simulink model "test_thrustflapping"  (Simulink 7.7)
settings: Solver=ode45  StartTime=0.0  StopTime=10  RelTol=1e-3
settings Model: Creator=Administrator  LastModifiedBy=Administrator
settings DataIOCC: LimitDataPoints=off  LoadExternalInput=on  OutputSaveName=T_MR

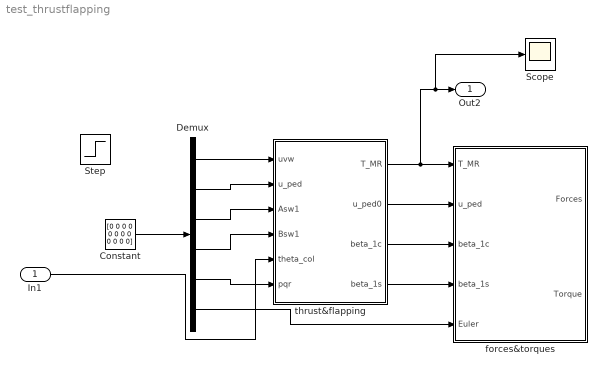
== system test_thrustflapping ==
  In1 : Inport
  Constant : Constant  Value=[0 0 0 0 0 0 0 0 0 0 0 0]
  Demux : Demux  Outputs=[3 1 1 1 3 3]
  Scope : Scope
  Step : Step  Time=0.5  After=0.5  SampleTime=0
  forces&torques : Subsystem  mask{mass0=44.384, AQ=0.00036, BQ=0.01, lm=0, ym=0, hm=0.2, Lt=1.2, Ht=0}
  thrust&flapping : Subsystem  mask{Ksw=0.2, Kcr=0.8, T_old=10, vi0=5, theta_twist=4.864e-4, theta_0=0.07}
  Out2 : Outport
  wires:
  Constant/1 -> Demux/1
  thrust&flapping/1(T_MR) -> forces&torques/1(T_MR), Out2/1, Scope/1
  thrust&flapping/2(u_ped0) -> forces&torques/2(u_ped)
  thrust&flapping/3(beta_1c) -> forces&torques/3(beta_1c)
  thrust&flapping/4(beta_1s) -> forces&torques/4(beta_1s)
  Demux/1 -> thrust&flapping/1(uvw)
  Demux/2 -> thrust&flapping/2(u_ped)
  Demux/3 -> thrust&flapping/3(Asw1)
  Demux/4 -> thrust&flapping/4(Bsw1)
  Demux/5 -> thrust&flapping/6(pqr)
  Demux/6 -> forces&torques/5(Euler)
  In1/1 -> thrust&flapping/5(theta_col)

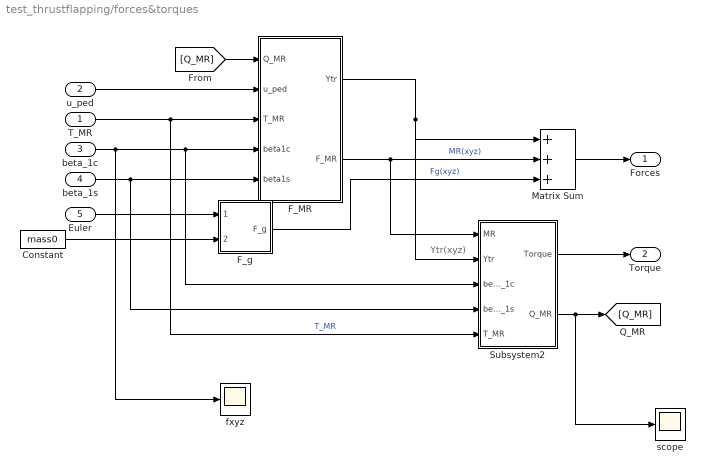
== system test_thrustflapping/forces&torques ==
  note: Ytr(xyz)
  T_MR : Inport
  u_ped : Inport  Port=2
  beta_1c : Inport  Port=3
  beta_1s : Inport  Port=4
  Euler : Inport  Port=5
  Constant : Constant  Value=mass0
  F_MR : Subsystem
  F_g : Subsystem
  Matrix Sum : Sum  Inputs=+++  CollapseMode=Specified dimension  CollapseDim=3
  Subsystem2 : Subsystem
  fxyz : Scope
      settings: YMin=-37.5  YMax=10  SaveName=ScopeData9
  scope : Scope
      settings: YMin=-37.5  YMax=10  SaveName=ScopeData14
  Forces : Outport
  Torque : Outport  Port=2
  wires:
  F_MR/1(Ytr) -> Subsystem2/2(Ytr), Matrix Sum/1
  u_ped/1 -> F_MR/2(u_ped)
  Matrix Sum/1 -> Forces/1
  Subsystem2/1(Torque) -> Torque/1
  Constant/1 -> F_g/2(mass)
  F_g/1(F_g) -> Matrix Sum/3  "Fg(xyz)"
  Euler/1 -> F_g/1(Euler)
  T_MR/1 -> Subsystem2/5(T_MR), F_MR/3(T_MR)  "T_MR"
  Subsystem2/2(Q_MR) -> [Q_MR], scope/1
  [Q_MR] -> F_MR/1(Q_MR)
  beta_1c/1 -> F_MR/4(beta1c), Subsystem2/3(beta_1c), fxyz/1
  beta_1s/1 -> F_MR/5(beta1s), Subsystem2/4(beta_1s)
  F_MR/2(F_MR) -> Subsystem2/1(MR), Matrix Sum/2  "MR(xyz)"

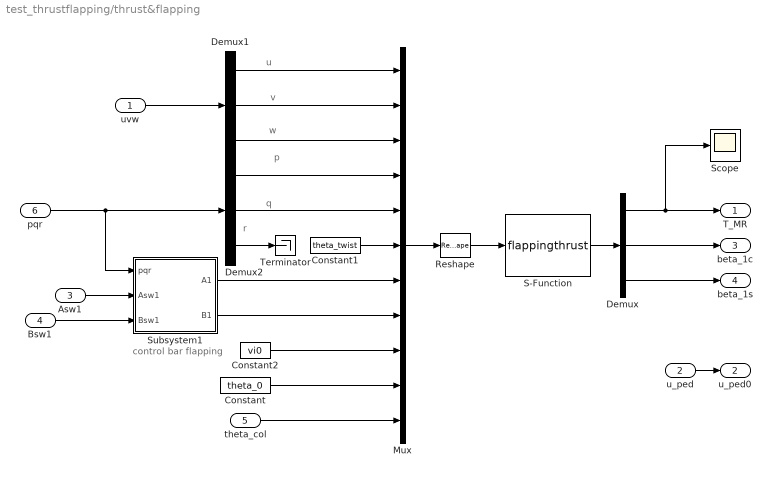
== system test_thrustflapping/thrust&flapping ==
  note: p
  note: q
  note: r
  note: u
  note: v
  note: w
  note: control bar flapping
  uvw : Inport
  u_ped : Inport  Port=2
  Asw1 : Inport  Port=3
  Bsw1 : Inport  Port=4
  theta_col : Inport  Port=5
  pqr : Inport  Port=6
  Constant : Constant  Value=theta_0
  Constant1 : Constant  Value=theta_twist
  Constant2 : Constant  Value=vi0
  Demux : Demux  Outputs=3
  Demux1 : Demux  Outputs=[1 1 1 ]
  Demux2 : Demux  Outputs=[1 1 1]
  Mux : Mux  Inputs=11
  Reshape : Reshape  OutputDimensionality=Column vector (2-D)
  S-Function : S-Function  RequirementInfo={} %GIDa_ec7bf881_92c1_4c8a_a396_57482acf355c  FunctionName=flappingthrust  EnableBusSupport=off
  Scope : Scope
      settings: SaveName=ScopeData4
  Subsystem1 : Subsystem
  Terminator : Terminator
  T_MR : Outport
  u_ped0 : Outport  Port=2
  beta_1c : Outport  Port=3
  beta_1s : Outport  Port=4
  wires:
  u_ped/1 -> u_ped0/1
  S-Function/1 -> Demux/1
  Demux/1 -> T_MR/1, Scope/1
  Demux/2 -> beta_1c/1
  Demux1/1 -> Mux/1
  Demux1/2 -> Mux/2
  Demux1/3 -> Mux/3
  uvw/1 -> Demux1/1
  Demux2/1 -> Mux/4
  Demux2/2 -> Mux/5
  pqr/1 -> Demux2/1, Subsystem1/1(pqr)
  Constant2/1 -> Mux/9
  Demux/3 -> beta_1s/1
  Constant/1 -> Mux/10
  Mux/1 -> Reshape/1
  Reshape/1 -> S-Function/1
  Asw1/1 -> Subsystem1/2(Asw1)
  Bsw1/1 -> Subsystem1/3(Bsw1)
  Subsystem1/1(A1) -> Mux/7
  Subsystem1/2(B1) -> Mux/8
  theta_col/1 -> Mux/11
  Demux2/3 -> Terminator/1
  Constant1/1 -> Mux/6

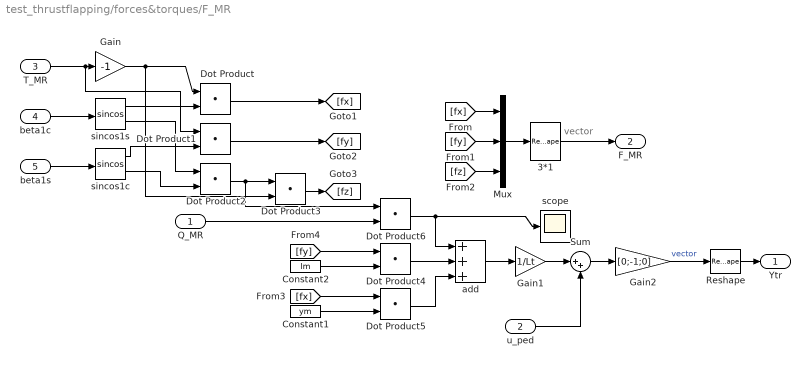
== system test_thrustflapping/forces&torques/F_MR ==
  note: vector
  Q_MR : Inport
  u_ped : Inport  Port=2
  T_MR : Inport  Port=3
  beta1c : Inport  Port=4
  beta1s : Inport  Port=5
  3*1 : Reshape  OutputDimensionality=Column vector (2-D)
  Constant1 : Constant  Value=ym
  Constant2 : Constant  Value=lm
  Dot Product{,1..6} (7 alike) : DotProduct  InputSameDT=on  OutDataTypeStr=Inherit: Inherit via internal rule
  Gain : Gain  Gain=-1
  Gain1 : Gain  Gain=1/Lt
  Gain2 : Gain  Gain=[0;-1;0]
  Mux : Mux  Inputs=3
  Reshape : Reshape  OutputDimensionality=Column vector (2-D)
  Sum : Sum  Inputs=|++
  add : Sum  Inputs=+++
  scope : Scope
      settings: YMin=-37.5  YMax=10  SaveName=ScopeData15
  sincos1c : Trigonometry  Operator=sincos
  sincos1s : Trigonometry  Operator=sincos
  Ytr : Outport
  F_MR : Outport  Port=2
  wires:
  u_ped/1 -> Sum/2
  Gain1/1 -> Sum/1
  add/1 -> Gain1/1
  Q_MR/1 -> Dot Product6/2
  Constant1/1 -> Dot Product5/2
  Constant2/1 -> Dot Product4/2
  Mux/1 -> 3*1/1
  beta1s/1 -> sincos1c/1
  beta1c/1 -> sincos1s/1
  Dot Product2/1 -> Dot Product6/1, Dot Product3/1
  sincos1c/2 -> Dot Product2/2
  sincos1s/2 -> Dot Product2/1
  sincos1c/1 -> Dot Product1/2
  sincos1s/1 -> Dot Product/2
  Gain/1 -> Dot Product3/2, Dot Product/1
  Dot Product/1 -> [fx]
  Dot Product1/1 -> [fy]
  Dot Product3/1 -> [fz]
  [fx] -> Mux/1
  [fy] -> Mux/2
  [fz] -> Mux/3
  [fy] -> Dot Product4/1
  [fx] -> Dot Product5/1
  Dot Product6/1 -> add/1, scope/1
  Dot Product4/1 -> add/2
  Dot Product5/1 -> add/3
  Sum/1 -> Gain2/1
  Gain2/1 -> Reshape/1  "vector"
  Reshape/1 -> Ytr/1
  3*1/1 -> F_MR/1
  T_MR/1 -> Dot Product1/1, Gain/1

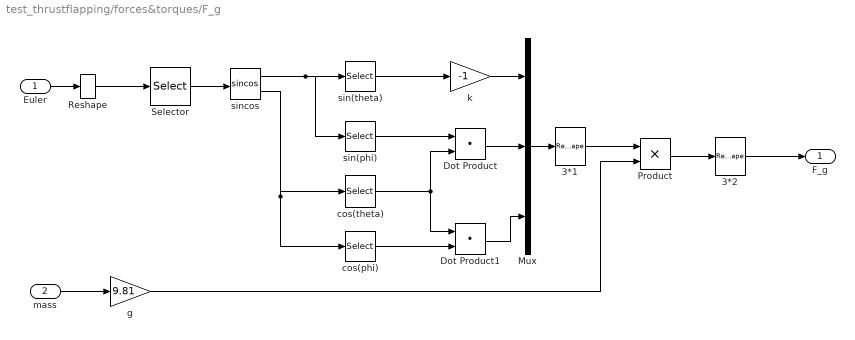
== system test_thrustflapping/forces&torques/F_g ==
  Euler : Inport
  mass : Inport  Port=2  PortDimensions=1
  3*1 : Reshape  OutputDimensionality=Column vector (2-D)
  3*2 : Reshape  OutputDimensionality=Column vector (2-D)
  Dot Product : DotProduct  InputSameDT=on  OutDataTypeStr=Inherit: Inherit via internal rule
  Dot Product1 : DotProduct  InputSameDT=on  OutDataTypeStr=Inherit: Inherit via internal rule
  Mux : Mux  Inputs=3
  Product : Product  RndMeth=Zero
  Reshape : Reshape  OutputDimensionality=Column vector (2-D)
  Selector : Selector  InputPortWidth=3  IndexOptions=Index vector (dialog)  Indices=[1 2]  OutputSizes=1
  cos(phi) : Selector  InputPortWidth=2  IndexOptions=Index vector (dialog)  Indices=[1]  OutputSizes=1
  cos(theta) : Selector  InputPortWidth=2  IndexOptions=Index vector (dialog)  Indices=[2]  OutputSizes=1
  g : Gain  Gain=9.81
  k : Gain  Gain=-1
  sin(phi) : Selector  InputPortWidth=2  IndexOptions=Index vector (dialog)  Indices=[1]  OutputSizes=1
  sin(theta) : Selector  InputPortWidth=2  IndexOptions=Index vector (dialog)  Indices=[2]  OutputSizes=1
  sincos : Trigonometry  Operator=sincos
  F_g : Outport
  wires:
  cos(phi)/1 -> Dot Product1/2
  Reshape/1 -> Selector/1
  Euler/1 -> Reshape/1
  mass/1 -> g/1
  Dot Product1/1 -> Mux/3
  Dot Product/1 -> Mux/2
  cos(theta)/1 -> Dot Product1/1, Dot Product/2
  sin(phi)/1 -> Dot Product/1
  k/1 -> Mux/1
  sin(theta)/1 -> k/1
  sincos/2 -> cos(theta)/1, cos(phi)/1
  sincos/1 -> sin(theta)/1, sin(phi)/1
  Selector/1 -> sincos/1
  Mux/1 -> 3*1/1
  3*1/1 -> Product/1
  g/1 -> Product/2
  Product/1 -> 3*2/1
  3*2/1 -> F_g/1

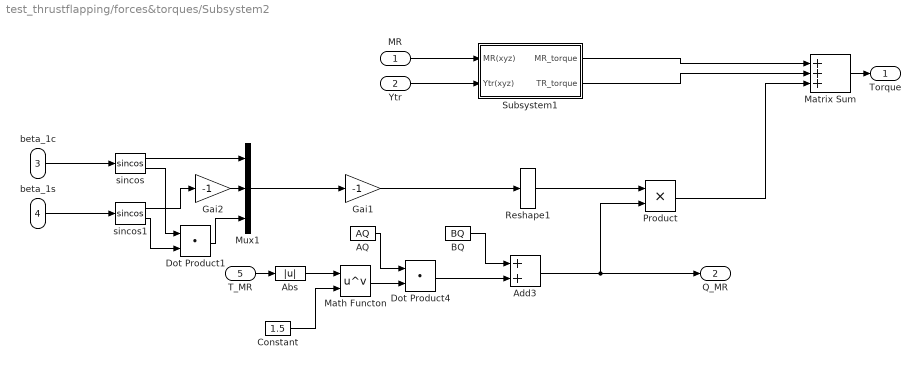
== system test_thrustflapping/forces&torques/Subsystem2 ==
  MR : Inport  PortDimensions=3
  Ytr : Inport  Port=2  PortDimensions=3
  beta_1c : Inport  Port=3  PortDimensions=1
  beta_1s : Inport  Port=4  PortDimensions=1
  T_MR : Inport  Port=5
  AQ : Constant  Value=AQ
  Abs : Abs
  Add3 : Sum
  BQ : Constant  Value=BQ  VectorParams1D=off
  Constant : Constant  Value=1.5
  Dot Product1 : DotProduct  InputSameDT=on  OutDataTypeStr=Inherit: Inherit via internal rule
  Dot Product4 : DotProduct  InputSameDT=on  OutDataTypeStr=Inherit: Inherit via internal rule
  Gai1 : Gain  Gain=-1
  Gai2 : Gain  Gain=-1
  Math Functon : Math  Operator=pow  SaturateOnIntegerOverflow=on
  Matrix Sum : Sum  Inputs=+++  CollapseMode=Specified dimension  CollapseDim=3
  Mux1 : Mux  Inputs=3
  Product : Product  RndMeth=Zero
  Reshape1 : Reshape  OutputDimensionality=Column vector (2-D)
  Subsystem1 : Subsystem
  sincos : Trigonometry  Operator=sincos
  sincos1 : Trigonometry  Operator=sincos
  Torque : Outport
  Q_MR : Outport  Port=2
  wires:
  Matrix Sum/1 -> Torque/1
  beta_1s/1 -> sincos1/1
  beta_1c/1 -> sincos/1
  Ytr/1 -> Subsystem1/2(Ytr(xyz))
  MR/1 -> Subsystem1/1(MR(xyz))
  Subsystem1/2(TR_torque) -> Matrix Sum/2
  Subsystem1/1(MR_torque) -> Matrix Sum/1
  Dot Product1/1 -> Mux1/3
  sincos/2 -> Dot Product1/1
  sincos1/2 -> Dot Product1/2
  Gai2/1 -> Mux1/2
  sincos1/1 -> Gai2/1
  sincos/1 -> Mux1/1
  Dot Product4/1 -> Add3/2
  BQ/1 -> Add3/1
  AQ/1 -> Dot Product4/1
  Math Functon/1 -> Dot Product4/2
  Constant/1 -> Math Functon/2
  Product/1 -> Matrix Sum/3
  Reshape1/1 -> Product/1
  T_MR/1 -> Abs/1
  Abs/1 -> Math Functon/1
  Add3/1 -> Product/2, Q_MR/1
  Mux1/1 -> Gai1/1
  Gai1/1 -> Reshape1/1

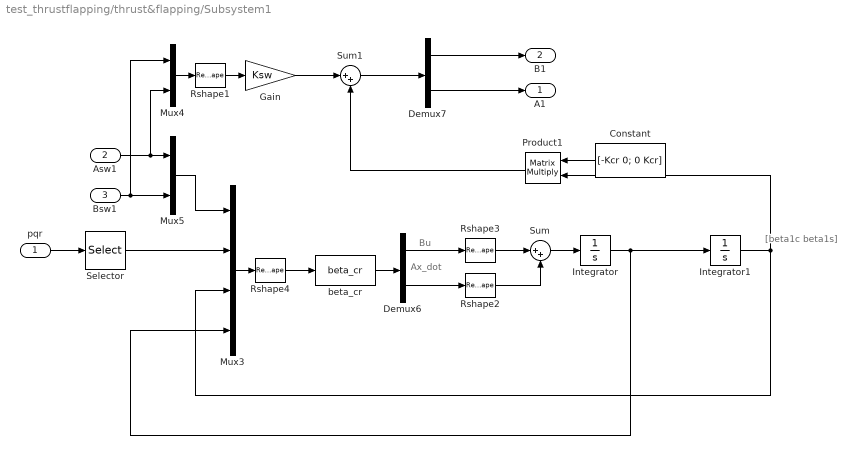
== system test_thrustflapping/thrust&flapping/Subsystem1 ==
  note: Ax_dot
  note: Bu
  note: [beta1c
      | beta1s]
  pqr : Inport
  Asw1 : Inport  Port=2
  Bsw1 : Inport  Port=3
  Constant : Constant  Value=[-Kcr 0; 0 Kcr]
  Demux6 : Demux  Outputs=[2 2]
  Demux7 : Demux  Outputs=[1 1]
  Gain : Gain  Gain=Ksw
  Integrator : Integrator  InitialCondition=[0;0]
  Integrator1 : Integrator  InitialCondition=[0;0]
  Mux3 : Mux
  Mux4 : Mux  Inputs=2
  Mux5 : Mux  Inputs=2
  Product1 : Product  Multiplication=Matrix(*)  RndMeth=Zero
  Rshape{1..4} (4 alike) : Reshape  OutputDimensionality=Column vector (2-D)
  Selector : Selector  InputPortWidth=3  IndexOptions=Index vector (dialog)  Indices=[1 2]  OutputSizes=1
  Sum : Sum  Inputs=|++
  Sum1 : Sum  Inputs=|++
  beta_cr : S-Function  FunctionName=beta_cr  EnableBusSupport=off
  A1 : Outport
  B1 : Outport  Port=2
  wires:
  Rshape4/1 -> beta_cr/1
  Mux3/1 -> Rshape4/1
  Rshape2/1 -> Sum/2
  Rshape3/1 -> Sum/1
  Demux6/2 -> Rshape2/1
  Demux6/1 -> Rshape3/1
  Selector/1 -> Mux3/2
  Mux5/1 -> Mux3/1
  pqr/1 -> Selector/1
  Product1/1 -> Sum1/2
  Mux4/1 -> Rshape1/1
  Rshape1/1 -> Gain/1
  Sum1/1 -> Demux7/1
  Gain/1 -> Sum1/1
  Constant/1 -> Product1/1
  Sum/1 -> Integrator/1
  beta_cr/1 -> Demux6/1
  Integrator1/1 -> Product1/2, Mux3/3
  Integrator/1 -> Integrator1/1, Mux3/4
  Bsw1/1 -> Mux5/2, Mux4/1
  Asw1/1 -> Mux5/1, Mux4/2
  Demux7/1 -> B1/1
  Demux7/2 -> A1/1

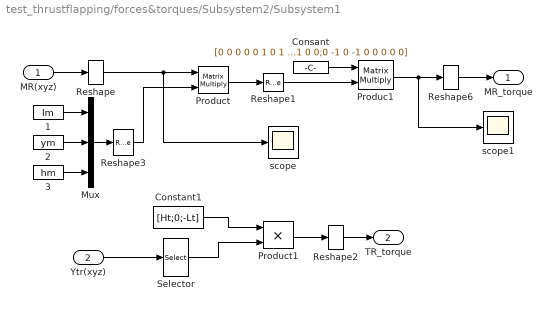
== system test_thrustflapping/forces&torques/Subsystem2/Subsystem1 ==
  MR(xyz) : Inport
  Ytr(xyz) : Inport  Port=2
  1 : Constant  Value=lm
  2 : Constant  Value=ym
  3 : Constant  Value=hm
  Consant : Constant  Value=[0 0 0 0 0 1 0 1 0;0 0 1 0 0 0 -1 0 0;0 -1 0 -1 0 0 0 0 0]
  Constant1 : Constant  Value=[Ht;0;-Lt]
  Mux : Mux  Inputs=3
  Produc1 : Product  Multiplication=Matrix(*)  RndMeth=Zero
  Product : Product  Multiplication=Matrix(*)  RndMeth=Zero
  Product1 : Product  RndMeth=Zero
  Reshape{,1..2,6} (4 alike) : Reshape  OutputDimensionality=Column vector (2-D)
  Reshape3 : Reshape  OutputDimensionality=Row vector (2-D)
  Selector : Selector  InputPortWidth=3  IndexOptions=Index vector (dialog)  Indices=[2]  OutputSizes=1
  scope : Scope
      settings: YMin=-37.5  YMax=10  SaveName=ScopeData10
  scope1 : Scope
      settings: YMin=-37.5  YMax=10  SaveName=ScopeData16
  MR_torque : Outport
  TR_torque : Outport  Port=2
  wires:
  Reshape6/1 -> MR_torque/1
  Produc1/1 -> Reshape6/1, scope1/1
  Consant/1 -> Produc1/1
  Reshape1/1 -> Produc1/2
  Ytr(xyz)/1 -> Selector/1
  Product/1 -> Reshape1/1
  Reshape3/1 -> Product/2
  Reshape/1 -> Product/1, scope/1
  Mux/1 -> Reshape3/1
  MR(xyz)/1 -> Reshape/1
  3/1 -> Mux/3
  2/1 -> Mux/2
  1/1 -> Mux/1
  Product1/1 -> Reshape2/1
  Reshape2/1 -> TR_torque/1
  Constant1/1 -> Product1/1
  Selector/1 -> Product1/2
